simulink library "lib_Chassis"  (R2017a)
settings: Solver=VariableStepAuto  StartTime=0.0  StopTime=10.0  RelTol=1e-3
undefined symbols (not defined in the file): g, Grade, mph2ms, rho, time, veh, Vehicle
settings Model: Creator=Di Russo  LastModifiedBy=Vraj M

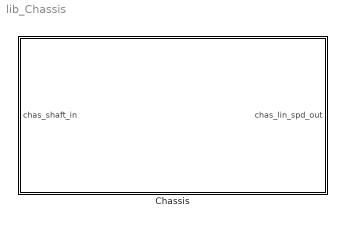
== system lib_Chassis ==
  Chassis : Subsystem
      mask Display:
      | image('Images/Chassis.JPG');
      | color('red');
      | port_label('input',1,'ShaftIn');
      | port_label('output',1,'SpdOut');

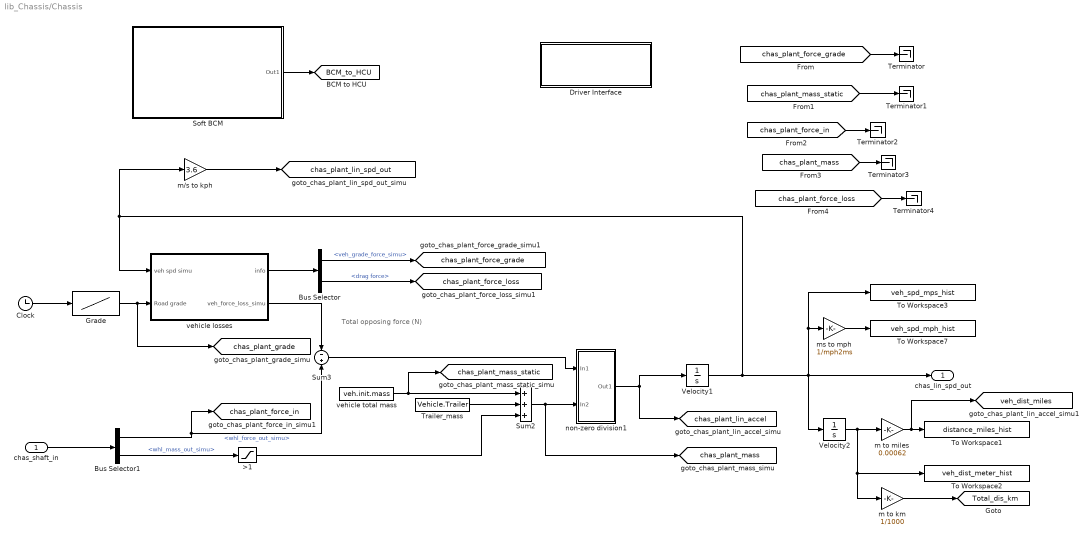
== system lib_Chassis/Chassis ==
  note: Total opposing
      | force (N)
  chas_shaft_in : Inport
  >1 : Saturate  UpperLimit=inf  LowerLimit=0
  Bus Selector : BusSelector  OutputSignals=veh_grade_force_simu,drag force
  Bus Selector1 : BusSelector  OutputSignals=whl_force_out_simu,whl_mass_out_simu
  Clock : Clock
  Driver Interface : Subsystem
  Grade : Lookup  InputValues=time  Table=Grade
  Soft BCM : Subsystem
      mask Display: image('SoftECU.jpg')
  Sum2 : Sum  Inputs=+++  SaturateOnIntegerOverflow=on  InputSameDT=on  OutDataTypeStr=Inherit: Same as first input
  Sum3 : Sum  Inputs=-+  SaturateOnIntegerOverflow=on  InputSameDT=on  OutDataTypeStr=Inherit: Same as first input
  Terminator{,1..4} (5 alike) : Terminator
  To Workspace1 : ToWorkspace  VariableName=distance_miles_hist  SampleTime=-1
      settings: Decimation=WORKSPACE_DECIMATION
  To Workspace2 : ToWorkspace  VariableName=veh_dist_meter_hist  SampleTime=-1
      settings: Decimation=WORKSPACE_DECIMATION
  To Workspace3 : ToWorkspace  VariableName=veh_spd_mps_hist  SampleTime=-1
      settings: Decimation=WORKSPACE_DECIMATION
  To Workspace7 : ToWorkspace  VariableName=veh_spd_mph_hist  SampleTime=-1
      settings: Decimation=WORKSPACE_DECIMATION
  Trailer_mass : Constant  Value=Vehicle.Trailer
  Velocity1 : Integrator  LimitOutput=on  LowerSaturationLimit=0
  Velocity2 : Integrator  LimitOutput=on  LowerSaturationLimit=0
  m to km : Gain  Gain=1/1000
  m to miles : Gain  Gain=0.00062
  m/s to kph : Gain  Gain=3.6
  ms to mph : Gain  Gain=1/mph2ms
  non-zero division1 : Subsystem
      mask Display: disp('divider \n I1/I2')
  vehicle losses : Subsystem
  vehicle total mass : Constant  Value=veh.init.mass
  chas_lin_spd_out : Outport
  tag scope: BCM_to_HCU=global, Total_dis_km=global, chas_plant_force_grade=global, chas_plant_force_in=global, chas_plant_force_loss=global, chas_plant_grade=global, chas_plant_lin_accel=global, chas_plant_lin_spd_out=global, chas_plant_mass=global, chas_plant_mass_static=global, veh_dist_miles=global
  wires:
  [chas_plant_force_loss] -> Terminator4/1
  [chas_plant_mass] -> Terminator3/1
  [chas_plant_force_in] -> Terminator2/1
  [chas_plant_mass_static] -> Terminator1/1
  [chas_plant_force_grade] -> Terminator/1
  Trailer_mass/1 -> Sum2/2
  m to km/1 -> [Total_dis_km]
  m to miles/1 -> To Workspace1/1, [veh_dist_miles]
  Velocity2/1 -> m to miles/1, m to km/1, To Workspace2/1
  Clock/1 -> Grade/1
  ms to mph/1 -> To Workspace7/1
  m/s to kph/1 -> [chas_plant_lin_spd_out]
  Soft BCM/1(Out1) -> [BCM_to_HCU]
  vehicle losses/2(veh_force_loss_simu) -> Sum3/1
  vehicle losses/1(info) -> Bus Selector/1
  chas_shaft_in/1 -> Bus Selector1/1
  Bus Selector1/1 -> [chas_plant_force_in], Sum3/2  "<whl_force_out_simu>"
  Bus Selector1/2 -> >1/1  "<whl_mass_out_simu>"
  >1/1 -> Sum2/3
  Sum2/1 -> [chas_plant_mass], non-zero division1/2(In2)
  Sum3/1 -> non-zero division1/1(In1)
  non-zero division1/1(Out1) -> [chas_plant_lin_accel], Velocity1/1
  Velocity1/1 -> chas_lin_spd_out/1, ms to mph/1, To Workspace3/1, Velocity2/1, m/s to kph/1, vehicle losses/1(veh spd simu)
  vehicle total mass/1 -> [chas_plant_mass_static], Sum2/1
  Bus Selector/1 -> [chas_plant_force_grade]  "<veh_grade_force_simu>"
  Bus Selector/2 -> [chas_plant_force_loss]  "<drag force>"
  Grade/1 -> [chas_plant_grade], vehicle losses/2(Road grade)

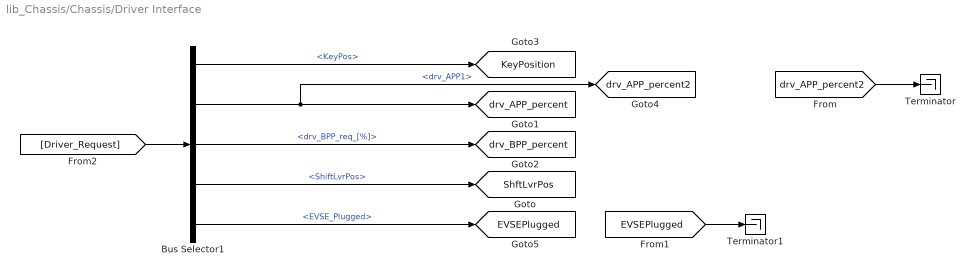
== system lib_Chassis/Chassis/Driver Interface ==
  Bus Selector1 : BusSelector  OutputSignals=KeyPos,drv_APP1,drv_BPP_req_[%],ShiftLvrPos,EVSE_Plugged
  Terminator : Terminator
  Terminator1 : Terminator
  tag scope: EVSEPlugged=global, KeyPosition=global, ShftLvrPos=global, drv_APP_percent2=global, drv_APP_percent=global, drv_BPP_percent=global
  wires:
  [EVSEPlugged] -> Terminator1/1
  [drv_APP_percent2] -> Terminator/1
  Bus Selector1/5 -> [EVSEPlugged]  "<EVSE_Plugged>"
  Bus Selector1/3 -> [drv_BPP_percent]  "<drv_BPP_req_[%]>"
  [Driver_Request] -> Bus Selector1/1
  Bus Selector1/4 -> [ShftLvrPos]  "<ShiftLvrPos>"
  Bus Selector1/2 -> [drv_APP_percent2], [drv_APP_percent]  "<drv_APP1>"
  Bus Selector1/1 -> [KeyPosition]  "<KeyPos>"

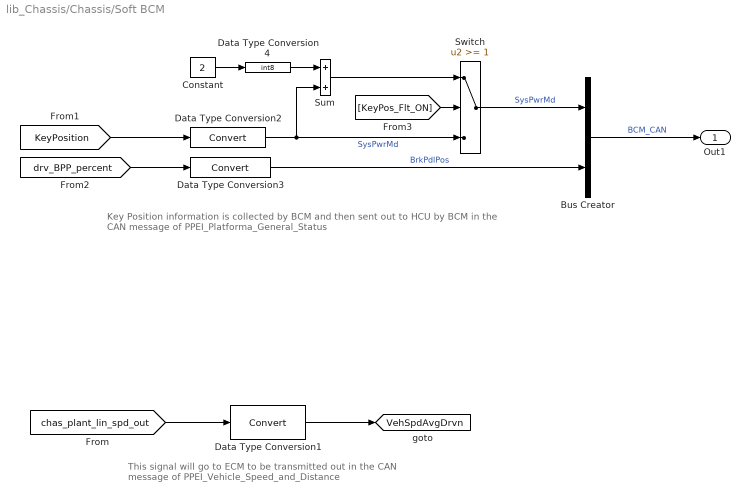
== system lib_Chassis/Chassis/Soft BCM ==
  note: Key Position information is collected by BCM and then sent out to HCU by BCM
      | in the CAN message of PPEI_Platforma_General_Status
  note: This signal will go to ECM to be transmitted out
      | in the CAN message of PPEI_Vehicle_Speed_and_Distance
  Bus Creator : BusCreator  Inputs=2
  Constant : Constant  Value=2
  Data Type Conversion1 : DataTypeConversion
  Data Type Conversion2 : DataTypeConversion
  Data Type Conversion3 : DataTypeConversion
  Data Type Conversion4 : DataTypeConversion  OutDataTypeStr=int8
  Sum : Sum
  Switch : Switch  Threshold=1
  Out1 : Outport
  tag scope: VehSpdAvgDrvn=global
  wires:
  Data Type Conversion4/1 -> Sum/1
  Constant/1 -> Data Type Conversion4/1
  Switch/1 -> Bus Creator/1  "SysPwrMd"
  Sum/1 -> Switch/1
  [KeyPos_Flt_ON] -> Switch/2
  Data Type Conversion3/1 -> Bus Creator/2  "BrkPdlPos"
  [drv_BPP_percent] -> Data Type Conversion3/1
  Bus Creator/1 -> Out1/1  "BCM_CAN"
  Data Type Conversion2/1 -> Sum/2, Switch/3  "SysPwrMd"
  [KeyPosition] -> Data Type Conversion2/1
  Data Type Conversion1/1 -> [VehSpdAvgDrvn]
  [chas_plant_lin_spd_out] -> Data Type Conversion1/1

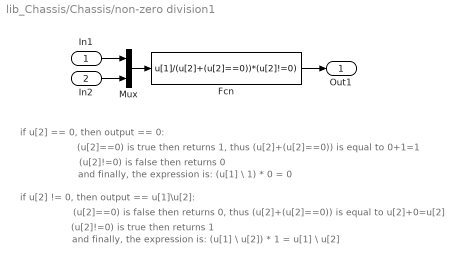
== system lib_Chassis/Chassis/non-zero division1 ==
  note: (u[2]==0) is true then returns 1, thus (u[2]+(u[2]==0)) is equal to 0+1=1
  note: if u[2] == 0, then output == 0:
  note: (u[2]!=0) is false then returns 0
  note: and finally, the expression is: (u[1] \ 1) * 0 = 0
  note: (u[2]==0) is false then returns 0, thus (u[2]+(u[2]==0)) is equal to u[2]+0=u[2]
  note: if u[2] != 0, then output == u[1]\u[2]:
  note: (u[2]!=0) is true then returns 1
  note: and finally, the expression is: (u[1] \ u[2]) * 1 = u[1] \ u[2]
  In1 : Inport
  In2 : Inport  Port=2
  Fcn : Fcn  Expr=u[1]/(u[2]+(u[2]==0))*(u[2]!=0)
  Mux : Mux  Inputs=2
  Out1 : Outport
  wires:
  Mux/1 -> Fcn/1
  In1/1 -> Mux/1
  Fcn/1 -> Out1/1
  In2/1 -> Mux/2

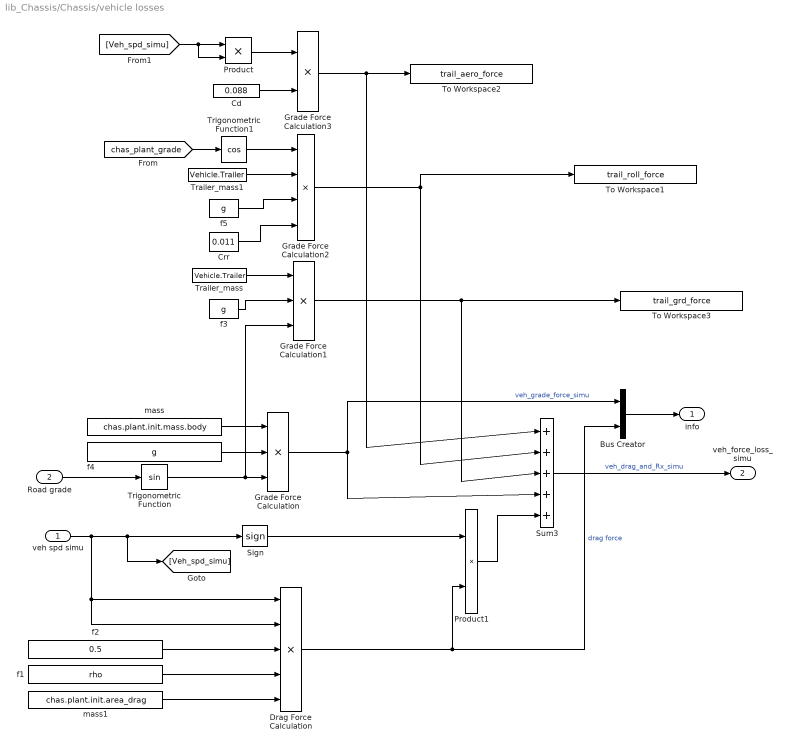
== system lib_Chassis/Chassis/vehicle losses ==
  veh spd simu : Inport
  Road grade : Inport  Port=2
  Bus Creator : BusCreator  Inputs=2
  Cd : Constant  Value=0.088
  Crr : Constant  Value=0.011
  Drag Force Calculation : Product  Inputs=5  SaturateOnIntegerOverflow=on  InputSameDT=on  OutDataTypeStr=Inherit: Same as first input
  Grade Force Calculation : Product  Inputs=3  SaturateOnIntegerOverflow=on  InputSameDT=on  OutDataTypeStr=Inherit: Same as first input
  Grade Force Calculation1 : Product  Inputs=3  SaturateOnIntegerOverflow=on  InputSameDT=on  OutDataTypeStr=Inherit: Same as first input
  Grade Force Calculation2 : Product  Inputs=4  SaturateOnIntegerOverflow=on  InputSameDT=on  OutDataTypeStr=Inherit: Same as first input
  Grade Force Calculation3 : Product  SaturateOnIntegerOverflow=on  InputSameDT=on  OutDataTypeStr=Inherit: Same as first input
  Product : Product
  Product1 : Product  SaturateOnIntegerOverflow=on  InputSameDT=on  OutDataTypeStr=Inherit: Same as first input
  Sign : Signum
  Sum3 : Sum  Inputs=|+++++  SaturateOnIntegerOverflow=on  InputSameDT=on  OutDataTypeStr=Inherit: Same as first input
  To Workspace1 : ToWorkspace  VariableName=trail_roll_force  SampleTime=-1
      settings: Decimation=WORKSPACE_DECIMATION
  To Workspace2 : ToWorkspace  VariableName=trail_aero_force  SampleTime=-1
      settings: Decimation=WORKSPACE_DECIMATION
  To Workspace3 : ToWorkspace  VariableName=trail_grd_force  SampleTime=-1
      settings: Decimation=WORKSPACE_DECIMATION
  Trailer_mass : Constant  Value=Vehicle.Trailer
  Trailer_mass1 : Constant  Value=Vehicle.Trailer
  Trigonometric Function : Trigonometry
  Trigonometric Function1 : Trigonometry  Operator=cos
  f1 : Constant  Value=rho
  f2 : Constant  Value=0.5
  f3 : Constant  Value=g
  f4 : Constant  Value=g
  f5 : Constant  Value=g
  mass : Constant  Value=chas.plant.init.mass.body
  mass1 : Constant  Value=chas.plant.init.area_drag
  info : Outport
  veh_force_loss_simu : Outport  Port=2
  wires:
  Grade Force Calculation3/1 -> To Workspace2/1, Sum3/1
  Cd/1 -> Grade Force Calculation3/2
  Product/1 -> Grade Force Calculation3/1
  [Veh_spd_simu] -> Product/1, Product/2
  Grade Force Calculation2/1 -> Sum3/2, To Workspace1/1
  Crr/1 -> Grade Force Calculation2/4
  f5/1 -> Grade Force Calculation2/3
  Trailer_mass1/1 -> Grade Force Calculation2/2
  Trigonometric Function1/1 -> Grade Force Calculation2/1
  Grade Force Calculation1/1 -> To Workspace3/1, Sum3/3
  f3/1 -> Grade Force Calculation1/2
  Trailer_mass/1 -> Grade Force Calculation1/1
  [chas_plant_grade] -> Trigonometric Function1/1
  f2/1 -> Drag Force Calculation/3
  mass1/1 -> Drag Force Calculation/5
  f1/1 -> Drag Force Calculation/4
  Trigonometric Function/1 -> Grade Force Calculation/3, Grade Force Calculation1/3
  f4/1 -> Grade Force Calculation/2
  mass/1 -> Grade Force Calculation/1
  Product1/1 -> Sum3/5
  Sign/1 -> Product1/1
  Road grade/1 -> Trigonometric Function/1
  Drag Force Calculation/1 -> Bus Creator/2, Product1/2  "drag force"
  veh spd simu/1 -> Drag Force Calculation/2, Drag Force Calculation/1, Sign/1, [Veh_spd_simu]
  Grade Force Calculation/1 -> Sum3/4, Bus Creator/1  "veh_grade_force_simu"
  Sum3/1 -> veh_force_loss_simu/1  "veh_drag_and_Rx_simu"
  Bus Creator/1 -> info/1
